simulink model "am"  (Simulink 5.0)
settings: Solver=ode45  StartTime=0.0  StopTime=10.0  RelTol=1e-3
settings Model: LastModifiedBy=Invitado

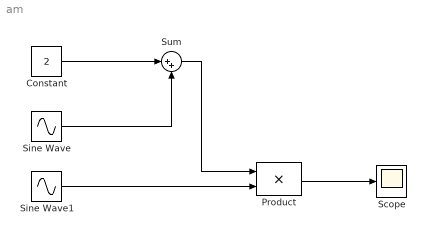
== system am ==
  Constant : Constant  Value=2
  Product : Product  SaturateOnIntegerOverflow=on
  Scope : Scope
      settings: TimeRange=10  SampleTime=0.01
  Sine Wave : Sin  Amplitude=2  SampleTime=0.01
  Sine Wave1 : Sin  Amplitude=2  Frequency=20  SampleTime=0.01
  Sum : Sum  Inputs=|++  SaturateOnIntegerOverflow=on
  wires:
  Constant/1 -> Sum/1
  Sine Wave/1 -> Sum/2
  Sum/1 -> Product/1
  Sine Wave1/1 -> Product/2
  Product/1 -> Scope/1
